simulink model "Regelkreis_begrenzt_windup"  (R2021a)
settings: Solver=VariableStepAuto  StartTime=0.0  StopTime=0.7  RelTol=1e-3
model workspace (MATLAB code in the model file):
  | T1 =  10 / 1000;
  | 
  | T2 = 100 / 1000;
  | 
  | Tn = 100 / 1000;
  | 
  | kp = 1;
  | 
  | v = 4;
  | 
  | w = 1;
  | 
  | u_max =  1.5;
  | u_min = -1.5;
  | 
  | y_max = v * u_max;
  | y_min = v * u_min;
  | 
  | T =   1 / 1000;
libraries: Regler x3
settings Model: OrderedModelArguments=off  Creator=Manoli  LastModifiedBy=Manoli

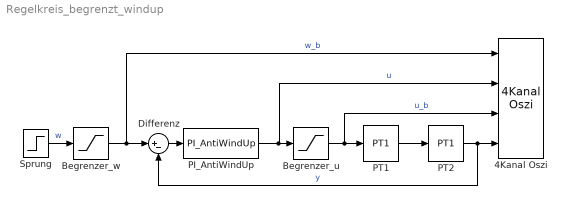
== system Regelkreis_begrenzt_windup ==
  4Kanal Oszi : Regler/4Kanal Oszi  N=20000  k=[1 1 1 1]  y=[-5 5]  tmax=1
  Begrenzer_u : Saturate  UpperLimit=u_max  LowerLimit=u_min
  Begrenzer_w : Saturate  UpperLimit=y_max  LowerLimit=y_min
  Differenz : Sum  Inputs=|+-  InputSameDT=on  SaturateOnIntegerOverflow=on  OutDataTypeStr=Inherit: Same as first input
  PI_AntiWindUp : S-Function  FunctionName=PI_AntiWindUp  Parameters=T  SFunctionDeploymentMode=off  EnableBusSupport=off
  PT1 : Regler/PT1  k=v  T1=T1
  PT2 : Regler/PT1  k=1  T1=T2
  Sprung : Step  Time=0.000001  After=w  SampleTime=0
  wires:
  PT1/1 -> PT2/1
  PT2/1 -> Differenz/2, 4Kanal Oszi/4  "y"
  Begrenzer_u/1 -> PT1/1, 4Kanal Oszi/3  "u_b"
  Differenz/1 -> PI_AntiWindUp/1
  Sprung/1 -> Begrenzer_w/1  "w"
  Begrenzer_w/1 -> Differenz/1, 4Kanal Oszi/1  "w_b"
  PI_AntiWindUp/1 -> 4Kanal Oszi/2, Begrenzer_u/1  "u"
